simulink model "CubeSatSimulation_Lite"  (R2024b)
settings: Solver=VariableStepAuto  StartTime=0.0  StopTime=100  RelTol=1e-3
values from neighbouring files (symbols this model uses):
  R = R_roll*R_pitch*R_yaw    [drawCubeSat.m]
undefined symbols (not defined in the file or in its folder): IAU, juliandate, sat, WMM2020
libraries: aerolibutil x6, matrix_library x6, simulink_extras x2, sharedutil x1, aerolibtransform2 x1, aerolibgravity2 x1, sharedtransform x1
settings Model: PacingRate=100  Creator=Ameya  LastModifiedBy=Ameya
settings RTWCC: GPUComputeCapability=3.5

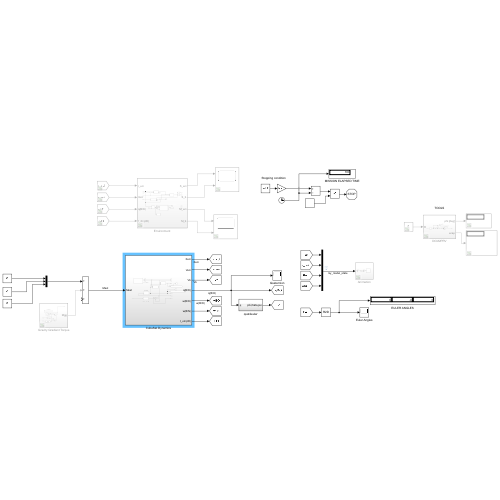
[thumbnail: Simulink's stored preview of the top-level diagram]
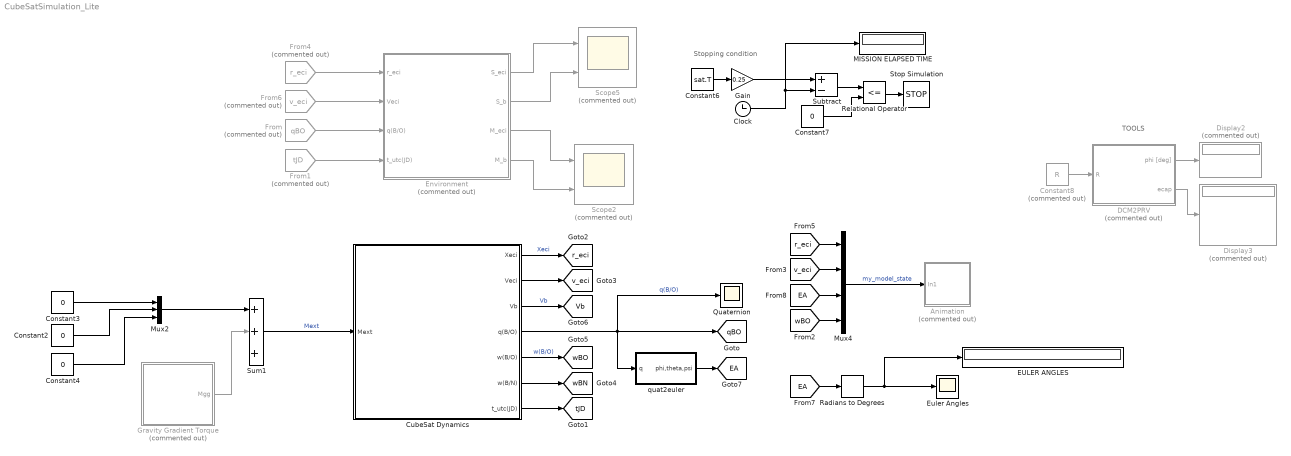
== system CubeSatSimulation_Lite ==
  note: TOOLS
  note: Stopping condition
  Animation : Subsystem  Commented=on
  Clock : Clock
  Constant{2..4,7} (4 alike) : Constant  Value=0
  Constant6 : Constant  Value=sat.T
  Constant8 : Constant  Commented=on  Value=R
  CubeSat Dynamics : Subsystem
  DCM2PRV : Subsystem  Commented=on
  Display2 : Display  Commented=on
  Display3 : Display  Commented=on
  EULER ANGLES : Display
  Environment : Subsystem  Commented=on
  Euler Angles : Scope
  From : From  Commented=on  GotoTag=qBO  TagVisibility=global
  From1 : From  Commented=on  GotoTag=tJD  TagVisibility=global
  From4 : From  Commented=on  GotoTag=r_eci  TagVisibility=global
  From6 : From  Commented=on  GotoTag=v_eci  TagVisibility=global
  Gain : Gain  Gain=0.25
  Gravity Gradient Torque : Subsystem  Commented=on
  MISSION ELAPSED TIME : Display
  Mux2 : Mux  Inputs=3
  Mux4 : Mux
  Quaternion : Scope
  Radians to Degrees : simulink_extras/Transformations/Radians to Degrees
  Relational Operator : RelationalOperator  Operator=<=  OutDataTypeStr=boolean  RndMeth=Simplest  InputSameDT=off
  Scope2 : Scope  Commented=on  NumInputPorts=2
  Scope5 : Scope  Commented=on  NumInputPorts=2
  Stop Simulation : Stop
  Subtract : Sum  Inputs=+-
  Sum1 : Sum  Inputs=+++
  quat2euler : Subsystem
  tag scope: EA=global, Vb=global, qBO=global, r_eci=global, tJD=global, v_eci=global, wBN=global, wBO=global
  wires:
  Constant3/1 -> Mux2/1
  Constant4/1 -> Mux2/3
  CubeSat Dynamics/4(q(B/O)) -> quat2euler/1(q), Quaternion/1, [qBO]  "q(B/O)"
  Mux4/1 -> Animation/1(In1)  "my_model_state"
  CubeSat Dynamics/5(w(B/O)) -> [wBO]  "w(B/O)"
  Environment/1(S_eci) -> Scope5/1
  CubeSat Dynamics/2(Veci) -> [v_eci]
  From/1 -> Environment/3(q(B/O))
  From1/1 -> Environment/4(t_utc(JD))
  Environment/2(S_b) -> Scope5/2
  CubeSat Dynamics/1(Xeci) -> [r_eci]  "Xeci"
  CubeSat Dynamics/7(t_utc(JD)) -> [tJD]
  Environment/3(M_eci) -> Scope2/1
  Environment/4(M_b) -> Scope2/2
  quat2euler/1(phi,theta,psi) -> [EA]
  Constant2/1 -> Mux2/2
  Mux2/1 -> Sum1/1
  Sum1/1 -> CubeSat Dynamics/1(Mext)  "Mext"
  Gravity Gradient Torque/1(Mgg) -> Sum1/2
  CubeSat Dynamics/6(w(B/N)) -> [wBN]
  [wBO] -> Mux4/4
  CubeSat Dynamics/3(Vb) -> [Vb]  "Vb"
  [v_eci] -> Mux4/2
  Radians to Degrees/1 -> EULER ANGLES/1, Euler Angles/1
  From4/1 -> Environment/1(r_eci)
  [r_eci] -> Mux4/1
  From6/1 -> Environment/2(Veci)
  [EA] -> Radians to Degrees/1
  [EA] -> Mux4/3
  Constant7/1 -> Relational Operator/2
  Constant6/1 -> Gain/1
  Clock/1 -> MISSION ELAPSED TIME/1, Subtract/2
  Gain/1 -> Subtract/1
  Subtract/1 -> Relational Operator/1
  Relational Operator/1 -> Stop Simulation/1
  Constant8/1 -> DCM2PRV/1(R)
  DCM2PRV/1(phi [deg]) -> Display2/1
  DCM2PRV/2(ecap) -> Display3/1

== system CubeSatSimulation_Lite/Animation ==
  In1 : Inport
  Clock : Clock
  CubeSat Attitude Animation : MATLABFcn  MATLABFcn=drawCubeSat  OutputDimensions=0
  Mux1 : Mux  Inputs=2
  wires:
  Mux1/1 -> CubeSat Attitude Animation/1
  In1/1 -> Mux1/1
  Clock/1 -> Mux1/2  "time"

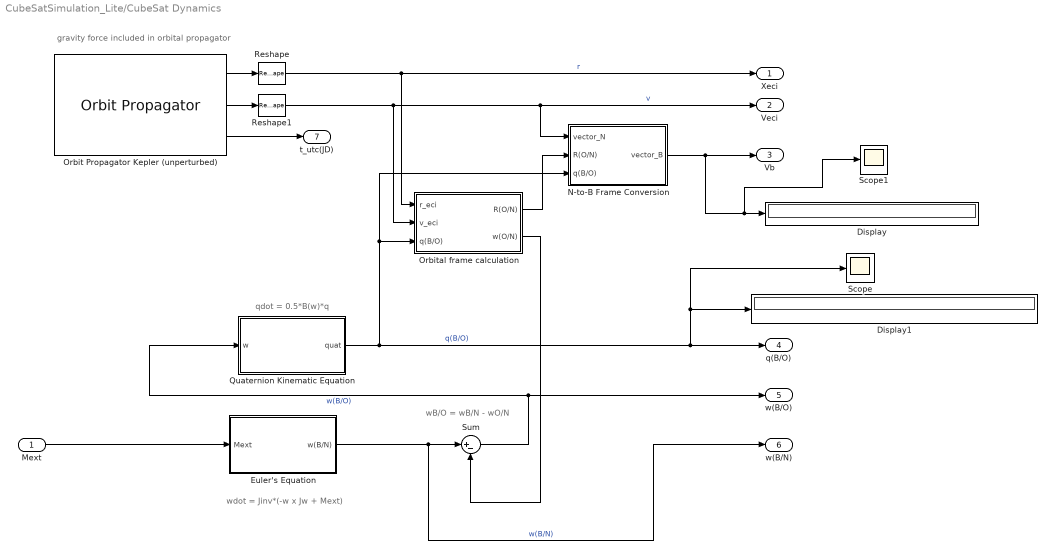
== system CubeSatSimulation_Lite/CubeSat Dynamics ==
  note: wB/O = wB/N - wO/N
  note: qdot = 0.5*B(w)*q
  note: wdot = Jinv*(-w x Jw + Mext)
  note: gravity force included in orbital propagator
  Mext : Inport
  Display : Display
  Display1 : Display
  Euler's Equation : Subsystem
  N-to-B Frame Conversion : Subsystem
  Orbit Propagator Kepler (unperturbed) : OrbitPropagator  accelIn=on  startDate=juliandate(2025, 1, 1, 12, 0, 0)  semiMajorAxis=sat.a  eccentricity=sat.e  inclination=rad2deg(sat.i)  raan=rad2deg(sat.RAAN)  argPeriapsis=rad2deg(sat.w)  trueAnomaly=rad2deg(sat.ta)  inertialPosition=[3649700.0 3308200.0 -4676600.0]  inertialVelocity=[-2750.8 6666.4 2573.4]  fixedPosition=[-4142689.0 -2676864.7 -4669861.6]  fixedVelocity=[1452.7 -6720.7 2568.1]  gravityModel=Oblate ellipsoid (J2)  customR=3396200  customMu=4.305e13  customJ2=1.0826269e-03  customOmega=4.06125949e-3
  Orbital frame calculation : Subsystem
  Quaternion Kinematic Equation : Subsystem
  Reshape : Reshape  OutputDimensionality=Column vector (2-D)
  Reshape1 : Reshape  OutputDimensionality=Column vector (2-D)
  Scope : Scope
  Scope1 : Scope
  Sum : Sum  Inputs=|+-
  Xeci : Outport
  Veci : Outport  Port=2
  Vb : Outport  Port=3
  q(B/O) : Outport  Port=4
  w(B/O) : Outport  Port=5
  w(B/N) : Outport  Port=6
  t_utc(JD) : Outport  Port=7
  wires:
  Mext/1 -> Euler's Equation/1(Mext)
  Euler's Equation/1(w(B/N)) -> w(B/N)/1, Sum/1  "w(B/N)"
  Sum/1 -> w(B/O)/1, Quaternion Kinematic Equation/1(w)  "w(B/O)"
  Orbital frame calculation/2(w(O/N)) -> Sum/2
  Quaternion Kinematic Equation/1(quat) -> N-to-B Frame Conversion/3(q(B/O)), Orbital frame calculation/3(q(B/O)), Display1/1, Scope/1, q(B/O)/1  "q(B/O)"
  Orbit Propagator Kepler (unperturbed)/1 -> Reshape/1
  Orbit Propagator Kepler (unperturbed)/2 -> Reshape1/1
  Reshape/1 -> Xeci/1, Orbital frame calculation/1(r_eci)  "r"
  Reshape1/1 -> N-to-B Frame Conversion/1(vector_N), Veci/1, Orbital frame calculation/2(v_eci)  "v"
  Orbital frame calculation/1(R(O/N)) -> N-to-B Frame Conversion/2(R(O/N))
  N-to-B Frame Conversion/1(vector_B) -> Scope1/1, Display/1, Vb/1
  Orbit Propagator Kepler (unperturbed)/3 -> t_utc(JD)/1

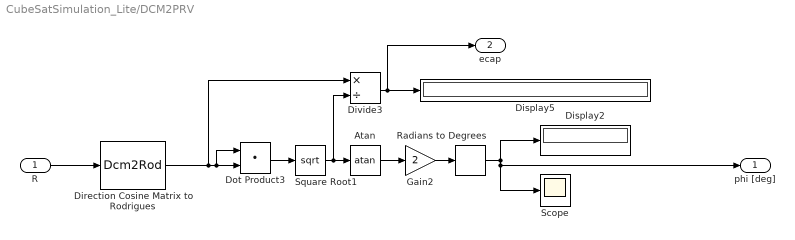
== system CubeSatSimulation_Lite/DCM2PRV ==
  R : Inport
  Atan : Trigonometry  Operator=atan
  Direction Cosine Matrix to Rodrigues : Dcm2Rod
  Display2 : Display
  Display5 : Display
  Divide3 : Product  Inputs=*/
  Dot Product3 : DotProduct  OutDataTypeStr=Inherit: Inherit via internal rule
  Gain2 : Gain  Gain=2
  Radians to Degrees : simulink_extras/Transformations/Radians to Degrees
  Scope : Scope
  Square Root1 : Sqrt
  phi [deg] : Outport
  ecap : Outport  Port=2
  wires:
  Radians to Degrees/1 -> phi [deg]/1, Scope/1, Display2/1
  Divide3/1 -> ecap/1, Display5/1
  R/1 -> Direction Cosine Matrix to Rodrigues/1
  Square Root1/1 -> Divide3/2, Atan/1
  Atan/1 -> Gain2/1
  Direction Cosine Matrix to Rodrigues/1 -> Divide3/1, Dot Product3/2, Dot Product3/1
  Dot Product3/1 -> Square Root1/1
  Gain2/1 -> Radians to Degrees/1

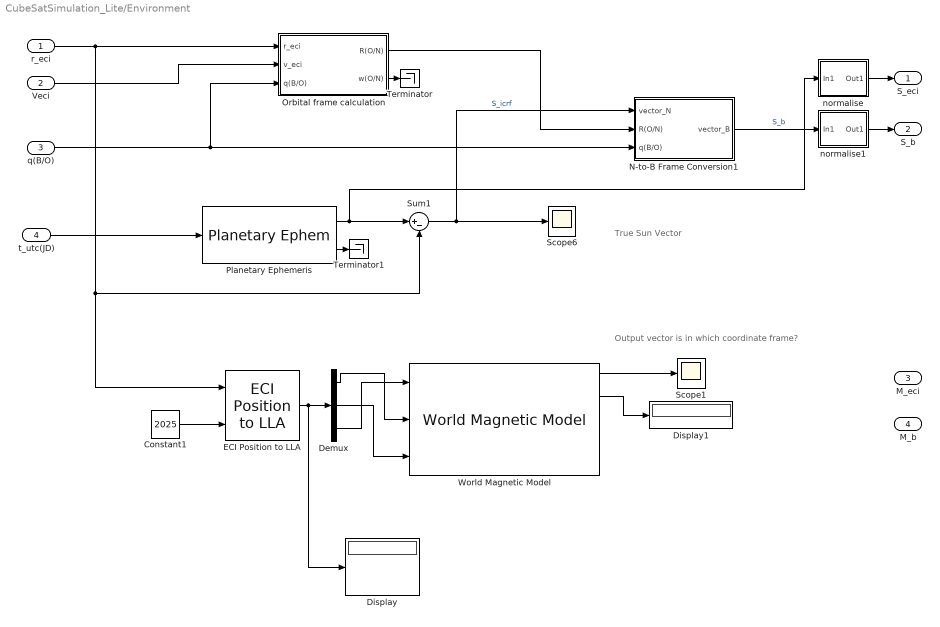
== system CubeSatSimulation_Lite/Environment ==
  note: Output vector is in which coordinate frame?
  note: True Sun Vector
  r_eci : Inport
  Veci : Inport  Port=2
  q(B/O) : Inport  Port=3
  t_utc(JD) : Inport  Port=4
  Constant1 : Constant  Value=2025
  Demux : Demux  Outputs=3
  Display : Display
  Display1 : Display
  ECI Position to LLA : aerolibtransform2/ECI Position to LLA  red=IAU-2000/2006  year=2025  month=January  day=1  hour=0  min=0  sec=0  deltaT=Day  errorflag=Error  extraparamflag=off  eunits=Metric (MKS)  earthmodel=WGS84  flat=1/298.257223563  eqradius=6378137
      settings: AttributesFormatString=%<red>
  N-to-B Frame Conversion1 : Subsystem
  Orbital frame calculation : Subsystem
  Planetary Ephemeris : PlanetaryEphem  target=Sun
  Scope1 : Scope
  Scope6 : Scope
  Sum1 : Sum  Inputs=|+-
  Terminator : Terminator
  Terminator1 : Terminator
  World Magnetic Model : aerolibgravity2/World Magnetic Model  model=WMM2020 (2020-2025)  customFile='WMM2020.COF'  units=Metric (MKS)  time_in=off  month=January  day=1  year=2020  action=Error  h_out=on  dec_out=on  inc_out=on  ti_out=on
  normalise : Subsystem
  normalise1 : Subsystem
  S_eci : Outport
  S_b : Outport  Port=2
  M_eci : Outport  Port=3
  M_b : Outport  Port=4
  wires:
  Orbital frame calculation/1(R(O/N)) -> N-to-B Frame Conversion1/2(R(O/N))
  Sum1/1 -> Scope6/1, N-to-B Frame Conversion1/1(vector_N)  "S_icrf"
  Planetary Ephemeris/1 -> Sum1/1, normalise/1(In1)
  q(B/O)/1 -> N-to-B Frame Conversion1/3(q(B/O)), Orbital frame calculation/3(q(B/O))
  r_eci/1 -> Sum1/2, ECI Position to LLA/1, Orbital frame calculation/1(r_eci)
  t_utc(JD)/1 -> Planetary Ephemeris/1
  N-to-B Frame Conversion1/1(vector_B) -> normalise1/1(In1)  "S_b"
  Planetary Ephemeris/2 -> Terminator1/1
  Orbital frame calculation/2(w(O/N)) -> Terminator/1
  Veci/1 -> Orbital frame calculation/2(v_eci)
  Demux/3 -> World Magnetic Model/1
  Demux/1 -> World Magnetic Model/2
  Demux/2 -> World Magnetic Model/3
  World Magnetic Model/1 -> Scope1/1
  Constant1/1 -> ECI Position to LLA/2
  ECI Position to LLA/1 -> Display/1, Demux/1
  World Magnetic Model/2 -> Display1/1
  normalise/1(Out1) -> S_eci/1
  normalise1/1(Out1) -> S_b/1

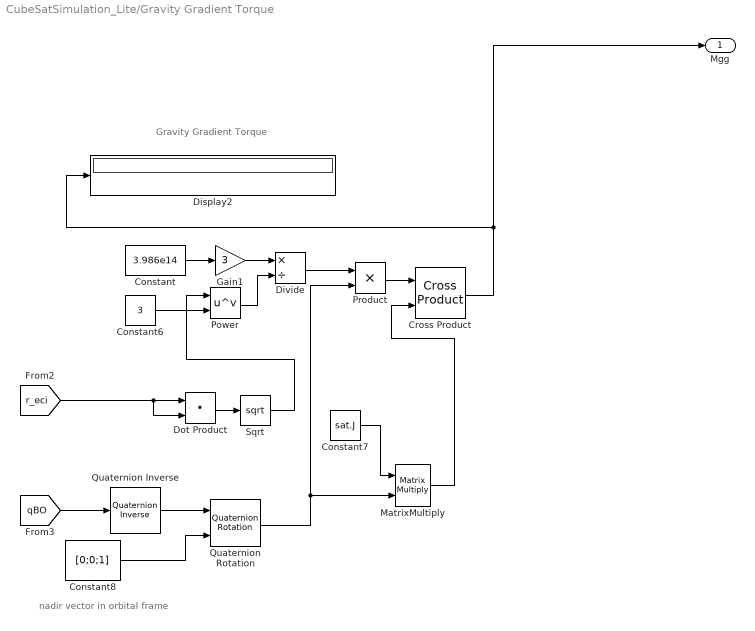
== system CubeSatSimulation_Lite/Gravity Gradient Torque ==
  note: Gravity Gradient Torque
  note: nadir vector in orbital frame
  Constant : Constant  Value=3.986e14
  Constant6 : Constant  Value=3
  Constant7 : Constant  Value=sat.J
  Constant8 : Constant  Value=[0;0;1]
  Cross Product : matrix_library/Cross Product
  Display2 : Display
  Divide : Product  Inputs=*/
  Dot Product : DotProduct  OutDataTypeStr=Inherit: Inherit via internal rule
  Gain1 : Gain  Gain=3
  MatrixMultiply : Product  Multiplication=Matrix(*)
  Power : Math  Operator=pow
  Product : Product
  Quaternion Inverse : aerolibutil/Quaternion Inverse
  Quaternion Rotation : aerolibutil/Quaternion Rotation
  Sqrt : Sqrt
  Mgg : Outport
  wires:
  Power/1 -> Divide/2
  Cross Product/1 -> Mgg/1, Display2/1
  MatrixMultiply/1 -> Cross Product/2
  Quaternion Inverse/1 -> Quaternion Rotation/1
  [qBO] -> Quaternion Inverse/1
  Sqrt/1 -> Power/1
  [r_eci] -> Dot Product/2, Dot Product/1
  Product/1 -> Cross Product/1
  Constant6/1 -> Power/2
  Dot Product/1 -> Sqrt/1
  Divide/1 -> Product/1
  Quaternion Rotation/1 -> Product/2, MatrixMultiply/2
  Gain1/1 -> Divide/1
  Constant/1 -> Gain1/1
  Constant8/1 -> Quaternion Rotation/2
  Constant7/1 -> MatrixMultiply/1

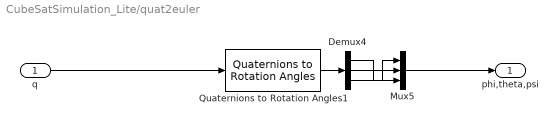
== system CubeSatSimulation_Lite/quat2euler ==
  q : Inport
  Demux4 : Demux  Outputs=3
  Mux5 : Mux  Inputs=3
  Quaternions to Rotation Angles1 : sharedtransform/Quaternions to Rotation Angles  rotationOrder=ZYX  aMode=aMode
  phi,theta,psi : Outport
  wires:
  Quaternions to Rotation Angles1/1 -> Demux4/1
  Demux4/3 -> Mux5/1
  Demux4/2 -> Mux5/2
  Demux4/1 -> Mux5/3
  q/1 -> Quaternions to Rotation Angles1/1
  Mux5/1 -> phi,theta,psi/1

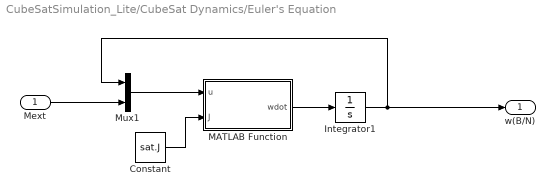
== system CubeSatSimulation_Lite/CubeSat Dynamics/Euler's Equation ==
  Mext : Inport
  Constant : Constant  Value=sat.J
  Integrator1 : Integrator  InitialCondition=sat.omegaBN
  MATLAB Function : MATLAB Function  TreatAsAtomicUnit=on
  Mux1 : Mux  Inputs=2
  w(B/N) : Outport
  wires:
  Mext/1 -> Mux1/2
  MATLAB Function/1(wdot) -> Integrator1/1
  Integrator1/1 -> Mux1/1, w(B/N)/1
  Mux1/1 -> MATLAB Function/1(u)
  Constant/1 -> MATLAB Function/2(J)

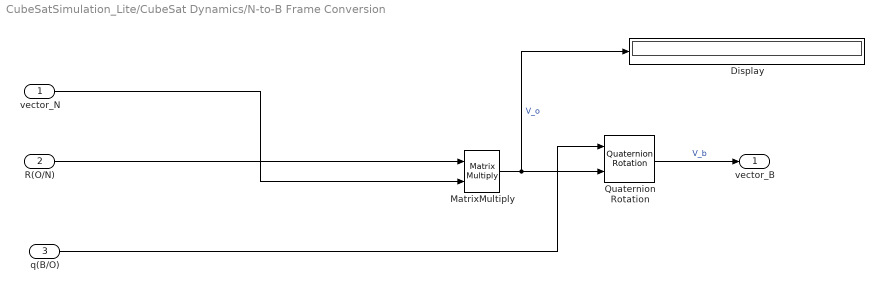
== system CubeSatSimulation_Lite/CubeSat Dynamics/N-to-B Frame Conversion ==
  vector_N : Inport
  R(O/N) : Inport  Port=2
  q(B/O) : Inport  Port=3
  Display : Display
  MatrixMultiply : Product  Multiplication=Matrix(*)
  Quaternion Rotation : aerolibutil/Quaternion Rotation
  vector_B : Outport
  wires:
  MatrixMultiply/1 -> Display/1, Quaternion Rotation/2  "V_o"
  Quaternion Rotation/1 -> vector_B/1  "V_b"
  R(O/N)/1 -> MatrixMultiply/1
  vector_N/1 -> MatrixMultiply/2
  q(B/O)/1 -> Quaternion Rotation/1

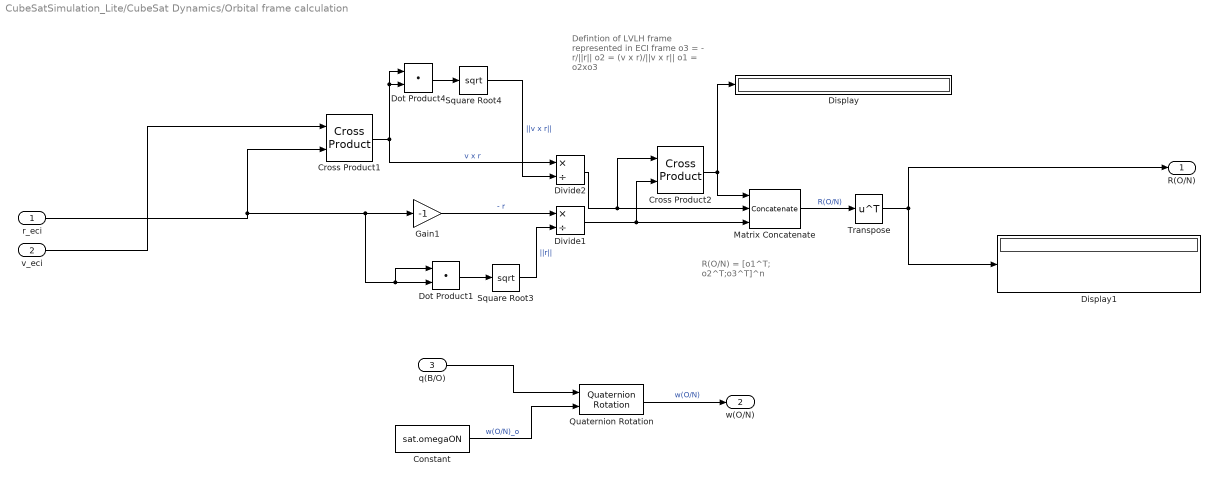
== system CubeSatSimulation_Lite/CubeSat Dynamics/Orbital frame calculation ==
  note: R(O/N) = [o1^T; o2^T;o3^T]^n
  note: Defintion of LVLH frame
      | represented in ECI frame
      | o3 = - r/||r||
      | o2 = (v x r)/||v x r||
      | o1 = o2xo3
  r_eci : Inport
  v_eci : Inport  Port=2
  q(B/O) : Inport  Port=3
  Constant : Constant  Value=sat.omegaON
  Cross Product1 : matrix_library/Cross Product
  Cross Product2 : matrix_library/Cross Product
  Display : Display
  Display1 : Display
  Divide1 : Product  Inputs=*/
  Divide2 : Product  Inputs=*/
  Dot Product1 : DotProduct  OutDataTypeStr=Inherit: Inherit via internal rule
  Dot Product4 : DotProduct  OutDataTypeStr=Inherit: Inherit via internal rule
  Gain1 : Gain  Gain=-1
  Matrix Concatenate : Concatenate  NumInputs=3  Mode=Multidimensional array  ConcatenateDimension=2
  Quaternion Rotation : aerolibutil/Quaternion Rotation
  Square Root3 : Sqrt
  Square Root4 : Sqrt
  Transpose : Math  Operator=transpose
  R(O/N) : Outport
  w(O/N) : Outport  Port=2
  wires:
  q(B/O)/1 -> Quaternion Rotation/1
  Quaternion Rotation/1 -> w(O/N)/1  "w(O/N)"
  Constant/1 -> Quaternion Rotation/2  "w(O/N)_o"
  Cross Product2/1 -> Display/1, Matrix Concatenate/1
  Divide2/1 -> Cross Product2/1, Matrix Concatenate/2
  Cross Product1/1 -> Dot Product4/2, Dot Product4/1, Divide2/1  "v x r"
  r_eci/1 -> Cross Product1/2, Dot Product1/1, Dot Product1/2, Gain1/1
  Gain1/1 -> Divide1/1  "- r"
  Square Root3/1 -> Divide1/2  "||r||"
  Square Root4/1 -> Divide2/2  "||v x r||"
  Dot Product1/1 -> Square Root3/1
  v_eci/1 -> Cross Product1/1
  Matrix Concatenate/1 -> Transpose/1  "R(O/N)"
  Divide1/1 -> Cross Product2/2, Matrix Concatenate/3
  Dot Product4/1 -> Square Root4/1
  Transpose/1 -> Display1/1, R(O/N)/1

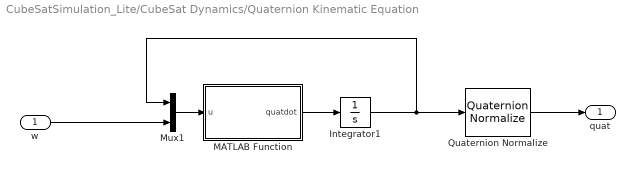
== system CubeSatSimulation_Lite/CubeSat Dynamics/Quaternion Kinematic Equation ==
  w : Inport
  Integrator1 : Integrator  InitialCondition=sat.quat
  MATLAB Function : MATLAB Function  TreatAsAtomicUnit=on
  Mux1 : Mux  Inputs=2
  Quaternion Normalize : sharedutil/Quaternion Normalize  aMode=aMode
  quat : Outport
  wires:
  Mux1/1 -> MATLAB Function/1(u)
  Integrator1/1 -> Quaternion Normalize/1, Mux1/1
  MATLAB Function/1(quatdot) -> Integrator1/1
  w/1 -> Mux1/2
  Quaternion Normalize/1 -> quat/1

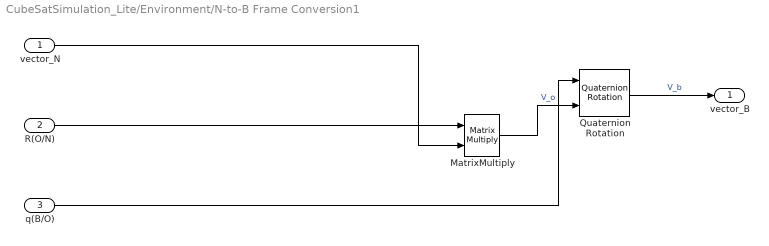
== system CubeSatSimulation_Lite/Environment/N-to-B Frame Conversion1 ==
  vector_N : Inport
  R(O/N) : Inport  Port=2
  q(B/O) : Inport  Port=3
  MatrixMultiply : Product  Multiplication=Matrix(*)
  Quaternion Rotation : aerolibutil/Quaternion Rotation
  vector_B : Outport
  wires:
  MatrixMultiply/1 -> Quaternion Rotation/2  "V_o"
  Quaternion Rotation/1 -> vector_B/1  "V_b"
  R(O/N)/1 -> MatrixMultiply/1
  vector_N/1 -> MatrixMultiply/2
  q(B/O)/1 -> Quaternion Rotation/1

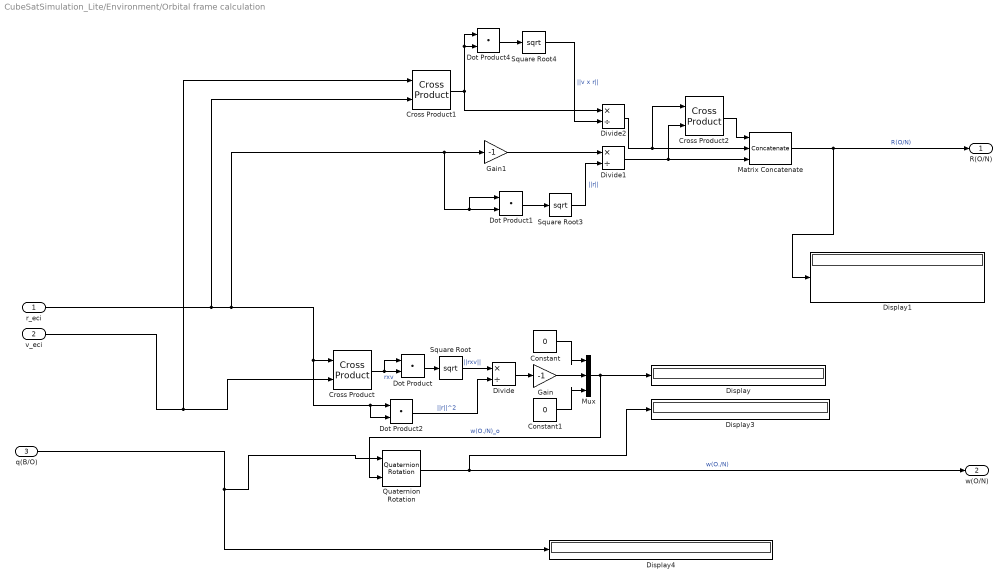
== system CubeSatSimulation_Lite/Environment/Orbital frame calculation ==
  r_eci : Inport
  v_eci : Inport  Port=2
  q(B/O) : Inport  Port=3
  Constant : Constant  Value=0
  Constant1 : Constant  Value=0
  Cross Product : matrix_library/Cross Product
  Cross Product1 : matrix_library/Cross Product
  Cross Product2 : matrix_library/Cross Product
  Display{,1,3..4} (4 alike) : Display
  Divide : Product  Inputs=*/
  Divide1 : Product  Inputs=*/
  Divide2 : Product  Inputs=*/
  Dot Product{,1..2,4} (4 alike) : DotProduct  OutDataTypeStr=Inherit: Inherit via internal rule
  Gain : Gain  Gain=-1
  Gain1 : Gain  Gain=-1
  Matrix Concatenate : Concatenate  NumInputs=3  Mode=Multidimensional array  ConcatenateDimension=2
  Mux : Mux  Inputs=3
  Quaternion Rotation : aerolibutil/Quaternion Rotation
  Square Root : Sqrt
  Square Root3 : Sqrt
  Square Root4 : Sqrt
  R(O/N) : Outport
  w(O/N) : Outport  Port=2
  wires:
  Constant1/1 -> Mux/3
  Dot Product2/1 -> Divide/2  "||r||^2"
  Gain/1 -> Mux/2
  q(B/O)/1 -> Display4/1, Quaternion Rotation/1
  Quaternion Rotation/1 -> Display3/1, w(O/N)/1  "w(O./N)"
  Cross Product/1 -> Dot Product/1, Dot Product/2  "rxv"
  Dot Product/1 -> Square Root/1
  Divide/1 -> Gain/1
  Square Root/1 -> Divide/1  "||rxv||"
  Mux/1 -> Quaternion Rotation/2, Display/1  "w(O./N)_o"
  Constant/1 -> Mux/1
  Cross Product2/1 -> Matrix Concatenate/1
  Divide2/1 -> Cross Product2/1, Matrix Concatenate/2
  Cross Product1/1 -> Dot Product4/2, Dot Product4/1, Divide2/1
  r_eci/1 -> Cross Product1/2, Dot Product1/1, Dot Product1/2, Gain1/1, Dot Product2/2, Dot Product2/1, Cross Product/1
  Gain1/1 -> Divide1/1
  Square Root3/1 -> Divide1/2  "||r||"
  Square Root4/1 -> Divide2/2  "||v x r||"
  Dot Product1/1 -> Square Root3/1
  v_eci/1 -> Cross Product1/1, Cross Product/2
  Matrix Concatenate/1 -> R(O/N)/1, Display1/1  "R(O/N)"
  Divide1/1 -> Cross Product2/2, Matrix Concatenate/3
  Dot Product4/1 -> Square Root4/1

== system CubeSatSimulation_Lite/Environment/normalise ==
  In1 : Inport
  Divide : Product  Inputs=*/
  Dot Product : DotProduct  OutDataTypeStr=Inherit: Inherit via internal rule
  Sqrt : Sqrt
  Out1 : Outport
  wires:
  Dot Product/1 -> Sqrt/1
  In1/1 -> Dot Product/2, Dot Product/1, Divide/1
  Divide/1 -> Out1/1
  Sqrt/1 -> Divide/2

== system CubeSatSimulation_Lite/Environment/normalise1 ==
  In1 : Inport
  Divide : Product  Inputs=*/
  Dot Product : DotProduct  OutDataTypeStr=Inherit: Inherit via internal rule
  Sqrt : Sqrt
  Out1 : Outport
  wires:
  Dot Product/1 -> Sqrt/1
  In1/1 -> Dot Product/2, Dot Product/1, Divide/1
  Divide/1 -> Out1/1
  Sqrt/1 -> Divide/2

== matlab function CubeSatSimulation_Lite/CubeSat Dynamics/Euler's Equation/MATLAB Function ==
  data: u input; wdot output; J input
function wdot = EulersEOM(u,J)
    w = u(1:3);
    m = u(4:6);
    wdot = J\(-cross(w,(J*w))+m);
end

== matlab function CubeSatSimulation_Lite/CubeSat Dynamics/Quaternion Kinematic Equation/MATLAB Function ==
  data: u input; quatdot output
function quatdot = quatKinematics(u)
    quat = u(1:4);
    p = u(5);
    q = u(6);
    r = u(7);
    quatdot = 0.5*[0,-p,-q,-r;
                p,0,r,-q;
                q,-r,0,p;
                r,q,-p,0]*quat;
end
